simulink model "flightplan"  (R2021b)
settings: Solver=VariableStepAuto  StartTime=0.0  StopTime=10.0  RelTol=1e-3
PreLoadFcn:
  | tabla1;
  | t2;
  | tabla3;
  | tablas.mat;
settings Model: Creator=verti  LastModifiedBy=verti
settings DataIOCC: ExternalInput=[DATA]  LoadExternalInput=on

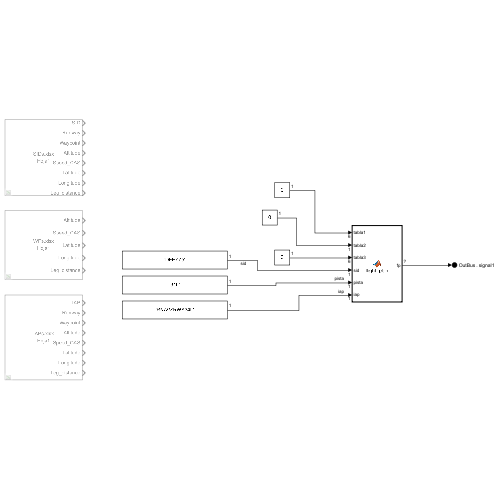
[thumbnail: Simulink's stored preview of the top-level diagram]
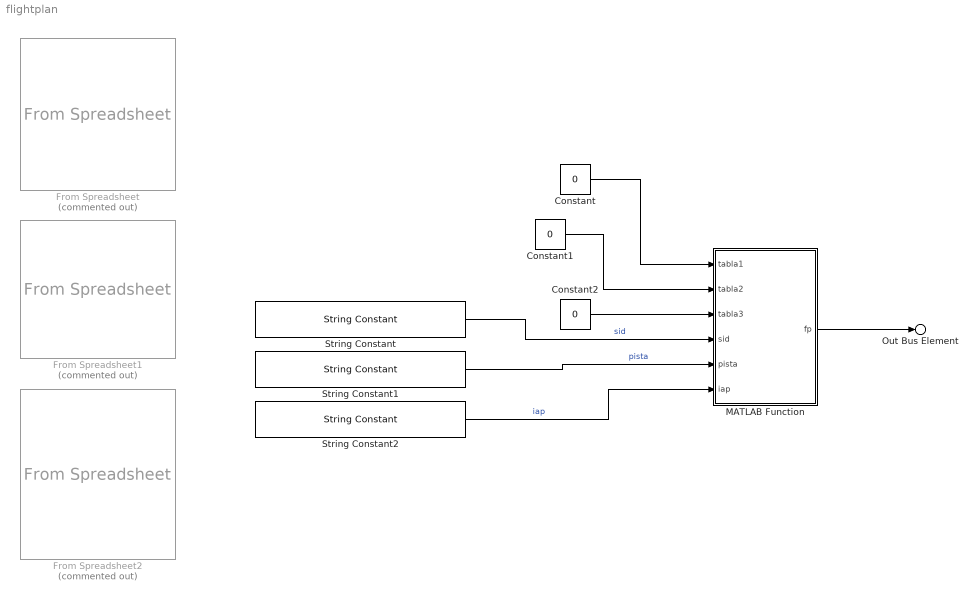
== system flightplan ==
  Constant : Constant  Value=0  OutDataTypeStr=Bus: BUS_SID
  Constant1 : Constant  Value=0  OutDataTypeStr=Bus: BUS_WP
  Constant2 : Constant  Value=0  OutDataTypeStr=Bus: BUS_IAP
  From Spreadsheet : FromSpreadsheet  Commented=on  FileName=SIDs.xlsx  SheetName=Hoja1
  From Spreadsheet1 : FromSpreadsheet  Commented=on  FileName=WPs.xlsx  SheetName=Hoja1
  From Spreadsheet2 : FromSpreadsheet  Commented=on  FileName=IAPs.xlsx  SheetName=Hoja1
  MATLAB Function : MATLAB Function  TreatAsAtomicUnit=on
  String Constant : StringConstant  String='DEEZZ5'
  String Constant1 : StringConstant  String='31L'
  String Constant2 : StringConstant  String='RNAVZRWY34L'
  Out Bus Element : Outport  PortName=OutBus  Element=signal1
  wires:
  String Constant1/1 -> MATLAB Function/5(pista)  "pista"
  String Constant/1 -> MATLAB Function/4(sid)  "sid"
  String Constant2/1 -> MATLAB Function/6(iap)  "iap"
  MATLAB Function/1(fp) -> Out Bus Element/1
  Constant1/1 -> MATLAB Function/2(tabla2)
  Constant/1 -> MATLAB Function/1(tabla1)
  Constant2/1 -> MATLAB Function/3(tabla3)

== matlab function flightplan/MATLAB Function ==
  data: tabla1 input; tabla2 input; tabla3 input; sid input; fp output; pista input; iap input
function fp  = flight_plan(tabla1,tabla2,tabla3,sid,pista,iap)

% Hay que proporcionarle 3 cadenas de carácteres SID,Pista de SID y el IAP.
% EJEMPLO: fp = flight_plan(tabla1,tabla2,tabla3,'DEEZZ5','22R','RNAVZRWY34L')

%% Antes de usar
%{
tabla1 = readtable('SIDs.xlsx');
tabla2 = readtable('WPs.xlsx');
tabla3 = readtable('IAPs.xlsx');
tabla1=table2struct(tabla1);
tabla2=table2struct(tabla2);
tabla3=table2struct(tabla3);
%}
%% Creación plan de vuelo (en tabla)

t111 = tabla1(strcmp({tabla1.SID},sid));
t11 = t111(strcmp({t111.Runway},pista));
t1 = rmfield(rmfield(rmfield(t11,'Airport'),'SID'),'Runway');
t33 = tabla3(strcmp({tabla3.IAP},iap));
t3 = rmfield(rmfield(rmfield(t33,'Airport'),'IAP'),'Runway');
fp=[t1;tabla2;t3];

%% Cálculo de distancias entre waypoints

for i=2:length(fp)
    fp(i).Leg_distance=60*distance('gc',fp(i).Latitude,fp(i).Longitude,fp(i-1).Latitude,fp(i-1).Longitude);
end


end
